simulink model "sim_3_twolink_task_control_ideal"  (R2021a)
settings: Solver=ode15s  StartTime=0.0  StopTime=20  RelTol=1e-5  EnableMultiTasking=on
values from neighbouring files (symbols this model uses):
  b1 = 0.01    [sim_params.m]    (also in sim_params_force.m)
  b2 = 0.01    [sim_params.m]    (also in sim_params_force.m)
  D = [zeros(n); eye(n)]    [control_comparison_script.m]    (also in gen_twolink_ss.m = reshape([0.0,0.0,0.0,0.0,0.0,0.0,0.0,0.0],[4,2]))
  D_T_Q = D'*Q    [control_comparison_script.m]
  epsilon = 0.1    [control_comparison_script.m]
  g = 9.80665    [sim_params.m]    (also in sim_params_force.m)
  Kpp = place(A,B,p)    [control_comparison_script.m]
  L1x = 0.3    [sim_params.m]    (also in sim_params_force.m)
  L1y = 0.050    (= 0.05)    [sim_params.m]    (also in sim_params_force.m)
  L1z = 0.05    [sim_params.m]    (also in sim_params_force.m)
  L2x = 0.15    [sim_params.m]    (also in sim_params_force.m = 0.3)
  L2y = 0.05    [sim_params.m]    (also in sim_params_force.m)
  L2z = 0.05    [sim_params.m]    (also in sim_params_force.m)
  m1 = m1*1.25    [control_comparison_script.m]    (also in sim_params.m = 2.775; sim_params_force.m = 2.775)
  m2 = m2*1.25    [control_comparison_script.m]    (also in sim_params.m = 1.3875; sim_params_force.m = 2.775)
  param_dev = 15    [control_comparison_script.m]
  rho = [1;1]    [control_comparison_script.m]
  theta1_0 = 0    [sim_params.m]    (also in sim_params_force.m = 1.57079632679)
  theta1_dot_0 = 0    [sim_params.m]    (also in sim_params_force.m)
  theta2_0 = 0    [sim_params.m]    (also in sim_params_force.m = -1.57079632679)
  theta2_dot_0 = 0    [sim_params.m]    (also in sim_params_force.m)
undefined symbols (not defined in the file or in its folder): Kd, Kd_grav, Kd_inv, Ki, Kp, Kp_grav, Kp_inv, N, sigbuilder_block, X, Y, Z
libraries: pid_lib x12, sm_lib x11, nesl_utility x10, spsFirstOrderFilterLib x4, dspmtrx3 x1, simulink x1
(part 1 of 3)
settings Model: Creator=bhorton  LastModifiedBy=Petronas-Tareq
settings SolverCC: ZeroCrossAlgorithm=Adaptive  AlgebraicLoopSolver=TrustRegion
settings DataIOCC: ReturnWorkspaceOutputs=off
settings OptimizationCC: LifeSpan=inf
settings DebuggingCC: SFUnexpectedBacktrackingDiag=warning  SFNoUnconditionalDefaultTransitionDiag=warning  SFExecutionAtInitializationDiag=none  SFMachineParentedDataDiag=warning  ArithmeticOperatorsInVariantConditions=warning
settings SFSimCC: SimUseLocalCustomCode=off  CustomCodeUndefinedFunction=UseInterfaceOnly
settings RTWCC: RTWUseLocalCustomCode=off
settings CodeAppCC: StateflowObjectComments=on
settings GRTTargetCC: TargetLangStandard=C89/C90 (ANSI)
settings ConfigComp: CovMetricSettings=dw  CovSaveCumulativeToWorkspaceVar=on  CovSaveSingleToWorkspaceVar=on  CovExternalEMLEnable=off
settings SimscapeCC: SimscapeNormalizeSystem=off  SimscapeLogType=all  SimscapeLogDataHistory=10000
settings ExplorerConfigSet: InternalSimMechanicsExplorerSettings="<ExplorerConfiguration><canonicalview>planar_xy</canonicalview><AnimationSetting><BasePlaybackSpeed>1.0</BasePlaybackSpeed><PlaybackSpeedFactor>4.0</PlaybackSpeedFactor></AnimationSetting><TilePanel><TileInfo><Tiles Columns=\"1\" Count=\"1\" Rows=\"1\"><Column Weight=\"1\"/><Row Weight=\"1\"/><Tile Height=\"1\" Width=\"1\" X=\"0\" Y=\"0\"/></Tiles></TileInfo><SceneInfo><SceneViewer><BGColor><R>0</R><G>0</G><B>0</B></BGColor><Camera><DoPerspective>off</DoPerspective><Position><X>0.0447898824465682299</X><Y>-0.016656403258507535</Y><Z>0.999999954328562035</Z></Position><Center><X>0.0447898824465682299</X><Y>-0.016656403258507535</Y><Z>-4.56714379648559543e-08</Z></Center><Up><X>0</X><Y>1</Y><Z>0</Z></Up><ViewLimDist>1</ViewLimDist><YLim>0.67213509984740738</YLim><XLim>1.22520332234454554</XLim></Camera></SceneViewer></SceneInfo></TilePanel><MechEditorPanel><Cameras/><GfxPanelCameraMap/><VideoCreator><PlaybackSpeedRatio>1</PlaybackSpeedRatio><FrameRate>30</FrameRate><VideoFormat>Motion JPEG AVI</VideoFormat><FrameSize>auto</FrameSize></VideoCreator></MechEditorPanel></ExplorerConfiguration>"

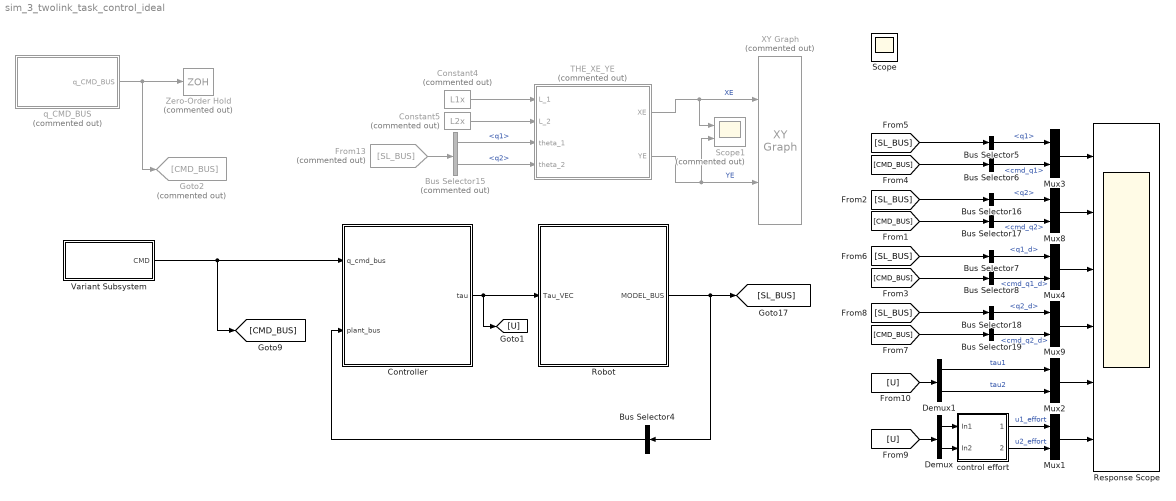
== system sim_3_twolink_task_control_ideal ==
  Bus Selector15 : BusSelector  Commented=on  OutputSignals=q1,q2
  Bus Selector16 : BusSelector  OutputSignals=q2
  Bus Selector17 : BusSelector  OutputSignals=cmd_q2
  Bus Selector18 : BusSelector  OutputSignals=q2_d
  Bus Selector19 : BusSelector  OutputSignals=cmd_q2_d
  Bus Selector4 : BusSelector  OutputSignals=q1_dd,q2_dd,q1_d,q2_d,q1,q2  OutputAsBus=on
  Bus Selector5 : BusSelector  OutputSignals=q1
  Bus Selector6 : BusSelector  OutputSignals=cmd_q1
  Bus Selector7 : BusSelector  OutputSignals=q1_d
  Bus Selector8 : BusSelector  OutputSignals=cmd_q1_d
  Constant4 : Constant  Commented=on  Value=L1x
  Constant5 : Constant  Commented=on  Value=L2x
  Controller : Subsystem  Variant=on  VariantControlMode=label  LabelModeActiveChoice=Inverse_dynamics_control  PropagateVariantConditions=on
  Demux : Demux  Outputs=2
  Demux1 : Demux  Outputs=2
  From13 : From  Commented=on  GotoTag=SL_BUS
  Goto2 : Goto  Commented=on  GotoTag=CMD_BUS
  Mux{1..4,8..9} (6 alike) : Mux  Inputs=2
  Response Scope : Scope  NumInputPorts=6
  Robot : Subsystem  Variant=on  VariantControlMode=label  LabelModeActiveChoice=Choice
  Scope1 : Scope  Commented=on  NumInputPorts=2
  THE_XE_YE : MATLAB Function  Commented=on  TreatAsAtomicUnit=on
  Variant Subsystem : Subsystem  Variant=on  VariantControlMode=label  LabelModeActiveChoice=Trapezoidal velocity
  XY Graph : simulink/Sinks/XY Graph  Commented=on  xmin=0  xmax=1.6  ymin=0  ymax=1.6  st=-1
  Zero-Order Hold : ZeroOrderHold  Commented=on  SampleTime=0.01
  control effort : Subsystem
  q_CMD_BUS : Subsystem  Commented=on
  Scope : Scope
  wires:
  [CMD_BUS] -> Bus Selector6/1
  [SL_BUS] -> Bus Selector5/1
  Mux3/1 -> Response Scope/1
  Bus Selector6/1 -> Mux3/2  "<cmd_q1>"
  Bus Selector5/1 -> Mux3/1  "<q1>"
  Bus Selector4/1 -> Controller/2(plant_bus)
  Mux4/1 -> Response Scope/3
  [SL_BUS] -> Bus Selector7/1
  [CMD_BUS] -> Bus Selector8/1
  Bus Selector8/1 -> Mux4/2  "<cmd_q1_d>"
  Bus Selector7/1 -> Mux4/1  "<q1_d>"
  Mux8/1 -> Response Scope/2
  [SL_BUS] -> Bus Selector16/1
  Bus Selector16/1 -> Mux8/1  "<q2>"
  [CMD_BUS] -> Bus Selector17/1
  Bus Selector17/1 -> Mux8/2  "<cmd_q2>"
  [CMD_BUS] -> Bus Selector19/1
  Mux9/1 -> Response Scope/4
  Bus Selector19/1 -> Mux9/2  "<cmd_q2_d>"
  Bus Selector18/1 -> Mux9/1  "<q2_d>"
  [SL_BUS] -> Bus Selector18/1
  Controller/1(tau) -> Robot/1(Tau_VEC), [U]
  [U] -> Demux/1
  Mux1/1 -> Response Scope/6
  Demux/1 -> control effort/1(In1)
  Demux/2 -> control effort/2(In2)
  control effort/1(u1_effort) -> Mux1/1  "u1_effort"
  control effort/2(u2_effort) -> Mux1/2  "u2_effort"
  [U] -> Demux1/1
  Mux2/1 -> Response Scope/5
  Demux1/1 -> Mux2/1  "tau1"
  Demux1/2 -> Mux2/2  "tau2"
  Variant Subsystem/1(CMD) -> [CMD_BUS], Controller/1(q_cmd_bus)
  Robot/1(MODEL_BUS) -> [SL_BUS], Bus Selector4/1
  From13/1 -> Bus Selector15/1
  Bus Selector15/2 -> THE_XE_YE/4(theta_2)  "<q2>"
  THE_XE_YE/2(YE) -> Scope1/2, XY Graph/2  "YE"
  Constant5/1 -> THE_XE_YE/2(L_2)
  Constant4/1 -> THE_XE_YE/1(L_1)
  THE_XE_YE/1(XE) -> Scope1/1, XY Graph/1  "XE"
  q_CMD_BUS/1(q_CMD_BUS) -> Goto2/1, Zero-Order Hold/1
  Bus Selector15/1 -> THE_XE_YE/3(theta_1)  "<q1>"

== system sim_3_twolink_task_control_ideal/Controller ==
  note: 1) Add Subsystem or Model blocks as valid variant choices.
      | 2) You cannot connect blocks at this level. At simulation, connectivity is automatically
      | determined, based on the active variant and port name matching.
  q_cmd_bus : Inport
  plant_bus : Inport  Port=2
  " Pole Placement Control" : Subsystem  VariantControl=PolePlacement_control
  "Inverse Dynamics control " : Subsystem  VariantControl=Inverse_dynamics_control
  PD Control : Subsystem  VariantControl=PD_control
  PD-feedforward-gravity Control : Subsystem  VariantControl=PD_feedforward_gravity
  "PD-gravity Control " : Subsystem  VariantControl=PD_plus_gravity
  PID Control : Subsystem  VariantControl=PID_control
  Pole Placement+D Control : Subsystem  VariantControl=PolePlacement_D_control
  "Robust control " : Subsystem  VariantControl=robust_control
  tau : Outport

== system sim_3_twolink_task_control_ideal/Robot ==
  note: 1) Add Subsystem or Model blocks as valid variant choices.
      | 2) You cannot connect blocks at this level. At simulation, connectivity is automatically
      | determined, based on the active variant and port name matching.
  Tau_VEC : Inport
  SIMSCAPE_MODEL : Subsystem  VariantControl=Choice_1
  SIMULINK_MODEL : Subsystem  VariantControl=Choice
  MODEL_BUS : Outport

== system sim_3_twolink_task_control_ideal/Variant Subsystem ==
  note: 1) Add Subsystem or Model blocks as valid variant choices.
      | 2) You cannot connect blocks at this level. At simulation, connectivity is automatically
      | determined, based on the active variant and port name matching.
  Sinewave command : Subsystem  VariantControl=sinwave
  Step command : Subsystem  VariantControl=step
  Trapezoidal velocity : Subsystem  VariantControl=Trapezoidal velocity
  CMD : Outport

== system sim_3_twolink_task_control_ideal/control effort ==
  In1 : Inport
  In2 : Inport  Port=2
  Integrator : Integrator
  Integrator1 : Integrator
  Square : Math  Operator=square  SaturateOnIntegerOverflow=on
  Square1 : Math  Operator=square  SaturateOnIntegerOverflow=on
  u1_effort : Outport
  u2_effort : Outport  Port=2
  wires:
  Square/1 -> Integrator/1
  Integrator1/1 -> u2_effort/1  "u2_effort"
  Integrator/1 -> u1_effort/1  "u1_effort"
  Square1/1 -> Integrator1/1
  In2/1 -> Square1/1
  In1/1 -> Square/1

== system sim_3_twolink_task_control_ideal/q_CMD_BUS ==
  Bus Creator : BusCreator  Inputs=4
  Bus Selector : BusSelector  OutputSignals=cmd_q1_d,cmd_q2_d,cmd_q1,cmd_q2
  From Spreadsheet : FromSpreadsheet  FileName=bh_2dof_q1_q2_for_hello.xlsx  SheetName=Q_for_hello  SampleTime=-1  ExtrapolationBeforeFirstDataPoint=Hold first value  ExtrapolationAfterLastDataPoint=Hold last value
  Scope : Scope  NumInputPorts=4
  q_CMD_BUS : Outport
  wires:
  From Spreadsheet/2 -> Bus Creator/2  "cmd_q2_d"
  From Spreadsheet/3 -> Bus Creator/3  "cmd_q1"
  From Spreadsheet/1 -> Bus Creator/1  "cmd_q1_d"
  From Spreadsheet/4 -> Bus Creator/4  "cmd_q2"
  Bus Creator/1 -> Bus Selector/1, q_CMD_BUS/1
  Bus Selector/1 -> Scope/1  "<cmd_q1_d>"
  Bus Selector/2 -> Scope/2  "<cmd_q2_d>"
  Bus Selector/3 -> Scope/3  "<cmd_q1>"
  Bus Selector/4 -> Scope/4  "<cmd_q2>"

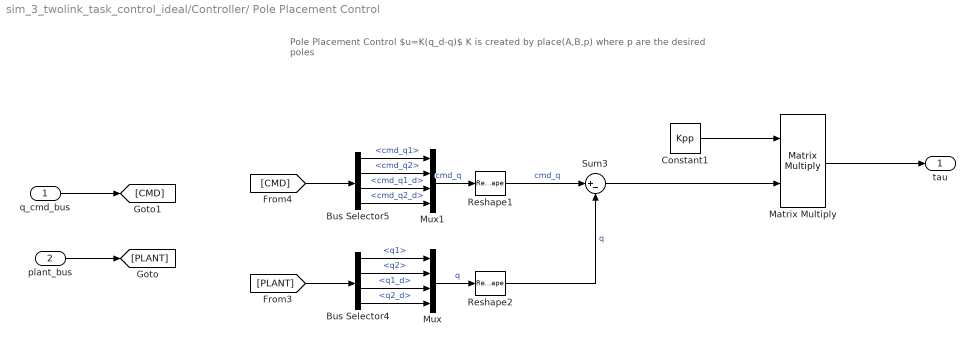
== system sim_3_twolink_task_control_ideal/Controller/ Pole Placement Control ==
  note: Pole Placement Control
      | $u=K(q_d-q)$
      | K is created by place(A,B,p) where p are the desired poles
  q_cmd_bus : Inport
  plant_bus : Inport  Port=2
  Bus Selector4 : BusSelector  OutputSignals=q1,q2,q1_d,q2_d
  Bus Selector5 : BusSelector  OutputSignals=cmd_q1,cmd_q2,cmd_q1_d,cmd_q2_d
  Constant1 : Constant  Value=Kpp  VectorParams1D=off
  Matrix Multiply : Product  Multiplication=Matrix(*)
  Mux : Mux
  Mux1 : Mux
  Reshape1 : Reshape  OutputDimensionality=Column vector (2-D)
  Reshape2 : Reshape  OutputDimensionality=Column vector (2-D)
  Sum3 : Sum  Inputs=|+-
  tau : Outport
  wires:
  plant_bus/1 -> [PLANT]
  q_cmd_bus/1 -> [CMD]
  [PLANT] -> Bus Selector4/1
  Bus Selector4/3 -> Mux/3  "<q1_d>"
  Bus Selector4/4 -> Mux/4  "<q2_d>"
  Mux/1 -> Reshape2/1  "q"
  Mux1/1 -> Reshape1/1  "cmd_q"
  [CMD] -> Bus Selector5/1
  Bus Selector5/3 -> Mux1/3  "<cmd_q1_d>"
  Bus Selector5/4 -> Mux1/4  "<cmd_q2_d>"
  Bus Selector5/2 -> Mux1/2  "<cmd_q2>"
  Bus Selector5/1 -> Mux1/1  "<cmd_q1>"
  Sum3/1 -> Matrix Multiply/2
  Reshape2/1 -> Sum3/2  "q"
  Reshape1/1 -> Sum3/1  "cmd_q"
  Constant1/1 -> Matrix Multiply/1
  Bus Selector4/1 -> Mux/1  "<q1>"
  Bus Selector4/2 -> Mux/2  "<q2>"
  Matrix Multiply/1 -> tau/1

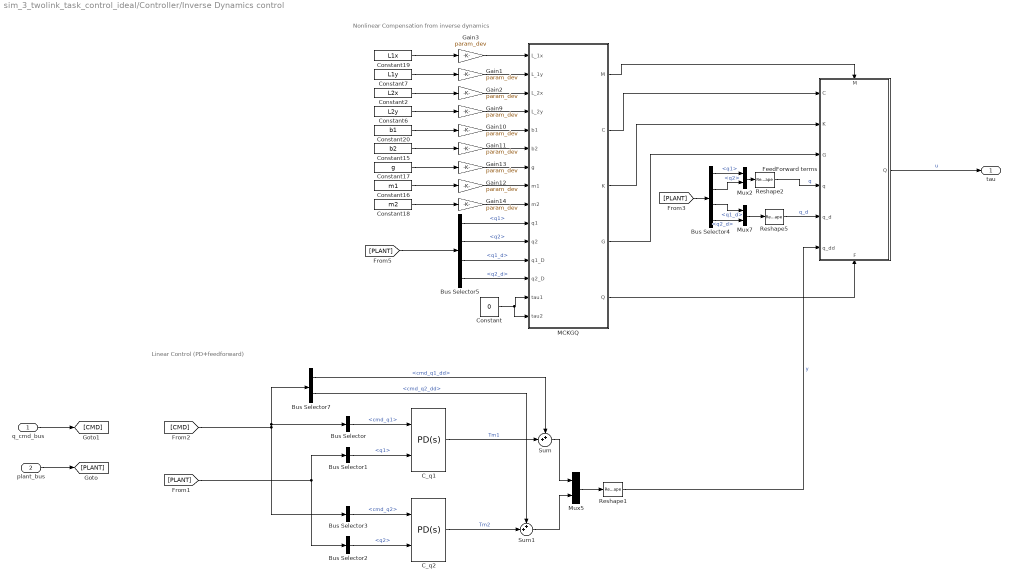
== system sim_3_twolink_task_control_ideal/Controller/Inverse Dynamics control  ==
  note: Nonlinear Compensation from inverse dynamics
  note: Linear Control (PD+feedforward)
  q_cmd_bus : Inport
  plant_bus : Inport  Port=2
  Bus Selector : BusSelector  OutputSignals=cmd_q1
  Bus Selector1 : BusSelector  OutputSignals=q1
  Bus Selector2 : BusSelector  OutputSignals=q2
  Bus Selector3 : BusSelector  OutputSignals=cmd_q2
  Bus Selector4 : BusSelector  OutputSignals=q1,q2,q1_d,q2_d
  Bus Selector5 : BusSelector  OutputSignals=q1,q2,q1_d,q2_d
  Bus Selector7 : BusSelector  OutputSignals=cmd_q1_dd,cmd_q2_dd
  C_q1 : pid_lib/PID Controller (2DOF)  Controller=PD  Form=Parallel  TimeDomain=Continuous-time  UseExternalTs=off  SampleTime=-1  IntegratorMethod=Forward Euler  FilterMethod=Forward Euler  ControllerParametersSource=internal  P=Kp_inv  I=20  D=Kd_inv  UseFilter=on  N=N  b=1  c=1  TunerSelectOption=Transfer Function Based (PID Tuner App)  InitialConditionSource=internal  InitialConditionForIntegrator=0  InitialConditionForFilter=0  DifferentiatorICPrevScaledInput=0  ExternalReset=none  TrackingMode=off  Kt=1  LimitOutput=off  SatLimitsSource=internal  UpperSaturationLimit=inf  LowerSaturationLimit=-inf  LinearizeAsGain=on  AntiWindupMode=none  Kb=1  POutMin=[]  POutMax=[]  IOutMin=[]  IOutMax=[]  DOutMin=[]  DOutMax=[]  NOutMin=[]  NOutMax=[]  bOutMin=[]  bOutMax=[]  cOutMin=[]  cOutMax=[]  SumOutMin=[]  SumOutMax=[]  SaturationOutMin=[]  SaturationOutMax=[]  PParamMin=[]  PParamMax=[]  IParamMin=[]  IParamMax=[]  DParamMin=[]  DParamMax=[]  NParamMin=[]  NParamMax=[]  bParamMin=[]  bParamMax=[]  cParamMin=[]  cParamMax=[]  KbParamMin=[]  KbParamMax=[]  KtParamMin=[]  KtParamMax=[]  KbOutMin=[]  KbOutMax=[]  KtOutMin=[]  KtOutMax=[]  IntegratorOutMin=[]  IntegratorOutMax=[]  FilterOutMin=[]  FilterOutMax=[]  SumI1OutMin=[]  SumI1OutMax=[]  SumI2OutMin=[]  SumI2OutMax=[]  SumI3OutMin=[]  SumI3OutMax=[]  SumI4OutMin=[]  SumI4OutMax=[]  SumDOutMin=[]  SumDOutMax=[]  Sum1OutMin=[]  Sum1OutMax=[]  Sum2OutMin=[]  Sum2OutMax=[]  Sum3OutMin=[]  Sum3OutMax=[]  DifferentiatorOutMin=[]  DifferentiatorOutMax=[]  FilterDiffOutCoefMin=[]  FilterDiffOutCoefMax=[]  ReciprocalOutMin=[]  ReciprocalOutMax=[]  SumDenOutMin=[]  SumDenOutMax=[]  SumNumOutMin=[]  SumNumOutMax=[]  DivideOutMin=[]  DivideOutMax=[]  UdiffTsProdOutMin=[]  UdiffTsProdOutMax=[]  NTsProdOutMin=[]  NTsProdOutMax=[]  UintegralTsProdOutMin=[]  UintegralTsProdOutMax=[]  UngainTsProdOutMin=[]  UngainTsProdOutMax=[]  IntegratorContinuousStateAttributes=''  IntegratorStateMustResolveToSignalObject=off  IntegratorRTWStateStorageClass=Auto  FilterContinuousStateAttributes=''  FilterStateMustResolveToSignalObject=off  FilterRTWStateStorageClass=Auto  ParallelPVariant=InternalParameters  IdealPVariant=Disabled  IVariant=Disabled  DVariant=InternalParameters  bVariant=InternalParameters  cVariant=InternalParameters  IntegratorVariant=Disabled  SatVariant=Disabled  AWVariant=Disabled  PCopyVariant=Disabled  TRVariant=Disabled  FdbkBlocksVariant=Forward  IdealPFdbkVariant=Disabled  SatFdbkVariant=Disabled  DerivativeFilterVariant=ContFilter  NVariant=InternalParameters  NCopyVariant=Disabled  FilterICVariant=InternalICsFilter  IntegratorICVariant=Disabled  ExternalResetVariant=Disabled  TRSumVariant=Passthrough  SumFdbkVariant=Disabled  SumVariant=Sum_PD  TsampFilterVariant=InternalTs  TsampNgainVariant=Passthrough  TsampIntegralVariant=Disabled_SignalSpec  ExternalSaturationOutDataTypeStr=Inherit: Same as second input
      settings: SourceProductBaseCode=SL
  C_q2 : pid_lib/PID Controller (2DOF)  Controller=PD  Form=Parallel  TimeDomain=Continuous-time  UseExternalTs=off  SampleTime=-1  IntegratorMethod=Forward Euler  FilterMethod=Forward Euler  ControllerParametersSource=internal  P=Kp_inv  I=20  D=Kd_inv  UseFilter=on  N=N  b=1  c=1  TunerSelectOption=Transfer Function Based (PID Tuner App)  InitialConditionSource=internal  InitialConditionForIntegrator=0  InitialConditionForFilter=0  DifferentiatorICPrevScaledInput=0  ExternalReset=none  TrackingMode=off  Kt=1  LimitOutput=off  SatLimitsSource=internal  UpperSaturationLimit=inf  LowerSaturationLimit=-inf  LinearizeAsGain=on  AntiWindupMode=none  Kb=1  POutMin=[]  POutMax=[]  IOutMin=[]  IOutMax=[]  DOutMin=[]  DOutMax=[]  NOutMin=[]  NOutMax=[]  bOutMin=[]  bOutMax=[]  cOutMin=[]  cOutMax=[]  SumOutMin=[]  SumOutMax=[]  SaturationOutMin=[]  SaturationOutMax=[]  PParamMin=[]  PParamMax=[]  IParamMin=[]  IParamMax=[]  DParamMin=[]  DParamMax=[]  NParamMin=[]  NParamMax=[]  bParamMin=[]  bParamMax=[]  cParamMin=[]  cParamMax=[]  KbParamMin=[]  KbParamMax=[]  KtParamMin=[]  KtParamMax=[]  KbOutMin=[]  KbOutMax=[]  KtOutMin=[]  KtOutMax=[]  IntegratorOutMin=[]  IntegratorOutMax=[]  FilterOutMin=[]  FilterOutMax=[]  SumI1OutMin=[]  SumI1OutMax=[]  SumI2OutMin=[]  SumI2OutMax=[]  SumI3OutMin=[]  SumI3OutMax=[]  SumI4OutMin=[]  SumI4OutMax=[]  SumDOutMin=[]  SumDOutMax=[]  Sum1OutMin=[]  Sum1OutMax=[]  Sum2OutMin=[]  Sum2OutMax=[]  Sum3OutMin=[]  Sum3OutMax=[]  DifferentiatorOutMin=[]  DifferentiatorOutMax=[]  FilterDiffOutCoefMin=[]  FilterDiffOutCoefMax=[]  ReciprocalOutMin=[]  ReciprocalOutMax=[]  SumDenOutMin=[]  SumDenOutMax=[]  SumNumOutMin=[]  SumNumOutMax=[]  DivideOutMin=[]  DivideOutMax=[]  UdiffTsProdOutMin=[]  UdiffTsProdOutMax=[]  NTsProdOutMin=[]  NTsProdOutMax=[]  UintegralTsProdOutMin=[]  UintegralTsProdOutMax=[]  UngainTsProdOutMin=[]  UngainTsProdOutMax=[]  IntegratorContinuousStateAttributes=''  IntegratorStateMustResolveToSignalObject=off  IntegratorRTWStateStorageClass=Auto  FilterContinuousStateAttributes=''  FilterStateMustResolveToSignalObject=off  FilterRTWStateStorageClass=Auto  ParallelPVariant=InternalParameters  IdealPVariant=Disabled  IVariant=Disabled  DVariant=InternalParameters  bVariant=InternalParameters  cVariant=InternalParameters  IntegratorVariant=Disabled  SatVariant=Disabled  AWVariant=Disabled  PCopyVariant=Disabled  TRVariant=Disabled  FdbkBlocksVariant=Forward  IdealPFdbkVariant=Disabled  SatFdbkVariant=Disabled  DerivativeFilterVariant=ContFilter  NVariant=InternalParameters  NCopyVariant=Disabled  FilterICVariant=InternalICsFilter  IntegratorICVariant=Disabled  ExternalResetVariant=Disabled  TRSumVariant=Passthrough  SumFdbkVariant=Disabled  SumVariant=Sum_PD  TsampFilterVariant=InternalTs  TsampNgainVariant=Passthrough  TsampIntegralVariant=Disabled_SignalSpec  ExternalSaturationOutDataTypeStr=Inherit: Same as second input
      settings: SourceProductBaseCode=SL
  Constant : Constant  Value=0
  Constant15 : Constant  Value=b2
  Constant16 : Constant  Value=m1
  Constant17 : Constant  Value=g
  Constant18 : Constant  Value=m2
  Constant19 : Constant  Value=L1x
  Constant2 : Constant  Value=L2x
  Constant20 : Constant  Value=b1
  Constant6 : Constant  Value=L2y
  Constant7 : Constant  Value=L1y
  FeedForward terms : Subsystem
      settings: PortSchema="{\"entries\":[{\"content\":{\"sides\":[{\"content\":{\"connectorIds\":[\"In1\",\"In2\",\"In3\",\"In4\",\"In5\",\"In6\"]},\"type\":\"ConnectorPlacement.EquallySpacedRectSide\",\"uuid\":\"236e7a2f-027c-4887-b3e9-bc0e11a59ec6\"},{\"content\":{\"connectorIds\":[\"Out1\"],\"side\":\"RIGHT\"},\"type\":\"ConnectorPlacement.EquallySpacedRectSide\",\"uuid\":\"0b727d96-7650-4ea0-95ac-5fb1bad7af10\"},{\"content\":{\"connectorIds\":[\"In7\"],\"side\":\"TOP\"},\"type\":\"ConnectorPlacement.EquallySpacedRectSide\",\"uuid\":\"19d9c8c6-ae7e-49b4-b718-472bd3040569\"},{\"content\":{\"connectorIds\":[\"In8\"],\"side\":\"BOTTOM\"},\"type\":\"ConnectorPlacement.EquallySpacedRectSide\",\"uuid\":\"734f5953-872d-4718-8798-69ea98da43e1\"}]},\"type\":\"ConnectorPlacement.EquallySpacedConnector\",\"uuid\":\"f4b93fea-e2dd-47f1-bf2a-cf2dec03adb9\"}],\"packageUris\":[\"http://schema.mathworks.com/mf0/Connector/R2020b\"],\"version\":\"1.0\"}"
  Gain{1..3,9..14} (9 alike) : Gain  Gain=param_dev
  MCKGQ : MATLAB Function  TreatAsAtomicUnit=on
  Mux2 : Mux  Inputs=2
  Mux5 : Mux  Inputs=2
  Mux7 : Mux  Inputs=2
  Reshape1 : Reshape  OutputDimensionality=Column vector (2-D)
  Reshape2 : Reshape  OutputDimensionality=Column vector (2-D)
  Reshape5 : Reshape  OutputDimensionality=Column vector (2-D)
  Sum : Sum  Inputs=++|
  Sum1 : Sum  Inputs=++|
  tau : Outport
  wires:
  C_q1/1 -> Sum/2  "Tm1"
  q_cmd_bus/1 -> [CMD]
  plant_bus/1 -> [PLANT]
  Bus Selector2/1 -> C_q2/2  "<q2>"
  Bus Selector3/1 -> C_q2/1  "<cmd_q2>"
  Bus Selector1/1 -> C_q1/2  "<q1>"
  Bus Selector/1 -> C_q1/1  "<cmd_q1>"
  [PLANT] -> Bus Selector1/1, Bus Selector2/1
  Constant17/1 -> Gain13/1
  Bus Selector5/4 -> MCKGQ/13(q2_D)  "<q2_d>"
  Constant16/1 -> Gain12/1
  Constant20/1 -> Gain10/1
  Constant2/1 -> Gain2/1
  Bus Selector5/3 -> MCKGQ/12(q1_D)  "<q1_d>"
  Bus Selector5/1 -> MCKGQ/10(q1)  "<q1>"
  Constant19/1 -> Gain3/1
  Constant15/1 -> Gain11/1
  Constant6/1 -> Gain9/1
  Constant7/1 -> Gain1/1
  Constant18/1 -> Gain14/1
  [PLANT] -> Bus Selector5/1
  Bus Selector5/2 -> MCKGQ/11(q2)  "<q2>"
  Mux5/1 -> Reshape1/1
  FeedForward terms/1(Q) -> tau/1  "u"
  [CMD] -> Bus Selector7/1, Bus Selector/1, Bus Selector3/1
  Bus Selector7/2 -> Sum1/1  "<cmd_q2_dd>"
  Sum/1 -> Mux5/1
  C_q2/1 -> Sum1/2  "Tm2"
  Sum1/1 -> Mux5/2
  [PLANT] -> Bus Selector4/1
  Bus Selector4/3 -> Mux7/1  "<q1_d>"
  Bus Selector4/4 -> Mux7/2  "<q2_d>"
  Mux7/1 -> Reshape5/1
  Reshape5/1 -> FeedForward terms/5(q_d)  "q_d"
  Reshape1/1 -> FeedForward terms/6(q_dd)  "y"
  MCKGQ/2(C) -> FeedForward terms/1(C)
  MCKGQ/3(K) -> FeedForward terms/2(K)
  MCKGQ/4(G) -> FeedForward terms/3(G)
  Bus Selector4/1 -> Mux2/1  "<q1>"
  Bus Selector4/2 -> Mux2/2  "<q2>"
  Mux2/1 -> Reshape2/1
  Reshape2/1 -> FeedForward terms/4(q)  "q"
  Bus Selector7/1 -> Sum/1  "<cmd_q1_dd>"
  MCKGQ/5(Q) -> FeedForward terms/8(F)
  Constant/1 -> MCKGQ/14(tau1), MCKGQ/15(tau2)
  MCKGQ/1(M) -> FeedForward terms/7(M)
  Gain1/1 -> MCKGQ/2(L_1y)
  Gain2/1 -> MCKGQ/3(L_2x)
  Gain9/1 -> MCKGQ/4(L_2y)
  Gain10/1 -> MCKGQ/5(b1)
  Gain11/1 -> MCKGQ/6(b2)
  Gain13/1 -> MCKGQ/7(g)
  Gain12/1 -> MCKGQ/8(m1)
  Gain14/1 -> MCKGQ/9(m2)
  Gain3/1 -> MCKGQ/1(L_1x)

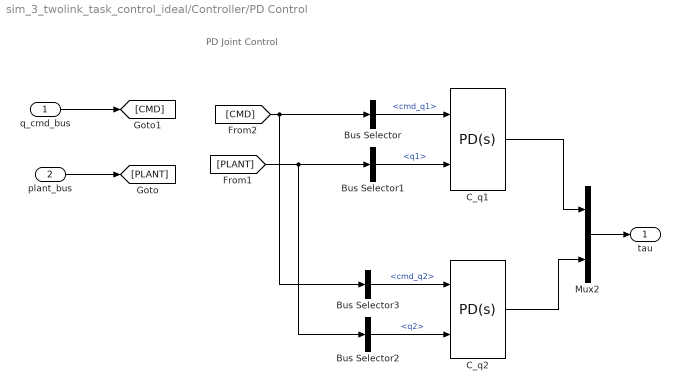
== system sim_3_twolink_task_control_ideal/Controller/PD Control ==
  note: PD Joint Control
  q_cmd_bus : Inport
  plant_bus : Inport  Port=2
  Bus Selector : BusSelector  OutputSignals=cmd_q1
  Bus Selector1 : BusSelector  OutputSignals=q1
  Bus Selector2 : BusSelector  OutputSignals=q2
  Bus Selector3 : BusSelector  OutputSignals=cmd_q2
  C_q1 : pid_lib/PID Controller (2DOF)  Controller=PD  Form=Parallel  TimeDomain=Continuous-time  UseExternalTs=off  SampleTime=-1  IntegratorMethod=Forward Euler  FilterMethod=Forward Euler  ControllerParametersSource=internal  P=Kp  I=20  D=Kd  UseFilter=on  N=N  b=1  c=1  TunerSelectOption=Transfer Function Based (PID Tuner App)  InitialConditionSource=internal  InitialConditionForIntegrator=0  InitialConditionForFilter=0  DifferentiatorICPrevScaledInput=0  ExternalReset=none  TrackingMode=off  Kt=1  LimitOutput=off  SatLimitsSource=internal  UpperSaturationLimit=inf  LowerSaturationLimit=-inf  LinearizeAsGain=on  AntiWindupMode=none  Kb=1  POutMin=[]  POutMax=[]  IOutMin=[]  IOutMax=[]  DOutMin=[]  DOutMax=[]  NOutMin=[]  NOutMax=[]  bOutMin=[]  bOutMax=[]  cOutMin=[]  cOutMax=[]  SumOutMin=[]  SumOutMax=[]  SaturationOutMin=[]  SaturationOutMax=[]  PParamMin=[]  PParamMax=[]  IParamMin=[]  IParamMax=[]  DParamMin=[]  DParamMax=[]  NParamMin=[]  NParamMax=[]  bParamMin=[]  bParamMax=[]  cParamMin=[]  cParamMax=[]  KbParamMin=[]  KbParamMax=[]  KtParamMin=[]  KtParamMax=[]  KbOutMin=[]  KbOutMax=[]  KtOutMin=[]  KtOutMax=[]  IntegratorOutMin=[]  IntegratorOutMax=[]  FilterOutMin=[]  FilterOutMax=[]  SumI1OutMin=[]  SumI1OutMax=[]  SumI2OutMin=[]  SumI2OutMax=[]  SumI3OutMin=[]  SumI3OutMax=[]  SumI4OutMin=[]  SumI4OutMax=[]  SumDOutMin=[]  SumDOutMax=[]  Sum1OutMin=[]  Sum1OutMax=[]  Sum2OutMin=[]  Sum2OutMax=[]  Sum3OutMin=[]  Sum3OutMax=[]  DifferentiatorOutMin=[]  DifferentiatorOutMax=[]  FilterDiffOutCoefMin=[]  FilterDiffOutCoefMax=[]  ReciprocalOutMin=[]  ReciprocalOutMax=[]  SumDenOutMin=[]  SumDenOutMax=[]  SumNumOutMin=[]  SumNumOutMax=[]  DivideOutMin=[]  DivideOutMax=[]  UdiffTsProdOutMin=[]  UdiffTsProdOutMax=[]  NTsProdOutMin=[]  NTsProdOutMax=[]  UintegralTsProdOutMin=[]  UintegralTsProdOutMax=[]  UngainTsProdOutMin=[]  UngainTsProdOutMax=[]  IntegratorContinuousStateAttributes=''  IntegratorStateMustResolveToSignalObject=off  IntegratorRTWStateStorageClass=Auto  FilterContinuousStateAttributes=''  FilterStateMustResolveToSignalObject=off  FilterRTWStateStorageClass=Auto  ParallelPVariant=InternalParameters  IdealPVariant=Disabled  IVariant=Disabled  DVariant=InternalParameters  bVariant=InternalParameters  cVariant=InternalParameters  IntegratorVariant=Disabled  SatVariant=Disabled  AWVariant=Disabled  PCopyVariant=Disabled  TRVariant=Disabled  FdbkBlocksVariant=Forward  IdealPFdbkVariant=Disabled  SatFdbkVariant=Disabled  DerivativeFilterVariant=ContFilter  NVariant=InternalParameters  NCopyVariant=Disabled  FilterICVariant=InternalICsFilter  IntegratorICVariant=Disabled  ExternalResetVariant=Disabled  TRSumVariant=Passthrough  SumFdbkVariant=Disabled  SumVariant=Sum_PD  TsampFilterVariant=InternalTs  TsampNgainVariant=Passthrough  TsampIntegralVariant=Disabled_SignalSpec  ExternalSaturationOutDataTypeStr=Inherit: Same as second input
      settings: SourceProductBaseCode=SL
  C_q2 : pid_lib/PID Controller (2DOF)  Controller=PD  Form=Parallel  TimeDomain=Continuous-time  UseExternalTs=off  SampleTime=-1  IntegratorMethod=Forward Euler  FilterMethod=Forward Euler  ControllerParametersSource=internal  P=Kp  I=307.702571204868  D=Kd  UseFilter=on  N=N  b=1  c=1  TunerSelectOption=Transfer Function Based (PID Tuner App)  InitialConditionSource=internal  InitialConditionForIntegrator=0  InitialConditionForFilter=0  DifferentiatorICPrevScaledInput=0  ExternalReset=none  TrackingMode=off  Kt=1  LimitOutput=off  SatLimitsSource=internal  UpperSaturationLimit=inf  LowerSaturationLimit=-inf  LinearizeAsGain=on  AntiWindupMode=none  Kb=1  POutMin=[]  POutMax=[]  IOutMin=[]  IOutMax=[]  DOutMin=[]  DOutMax=[]  NOutMin=[]  NOutMax=[]  bOutMin=[]  bOutMax=[]  cOutMin=[]  cOutMax=[]  SumOutMin=[]  SumOutMax=[]  SaturationOutMin=[]  SaturationOutMax=[]  PParamMin=[]  PParamMax=[]  IParamMin=[]  IParamMax=[]  DParamMin=[]  DParamMax=[]  NParamMin=[]  NParamMax=[]  bParamMin=[]  bParamMax=[]  cParamMin=[]  cParamMax=[]  KbParamMin=[]  KbParamMax=[]  KtParamMin=[]  KtParamMax=[]  KbOutMin=[]  KbOutMax=[]  KtOutMin=[]  KtOutMax=[]  IntegratorOutMin=[]  IntegratorOutMax=[]  FilterOutMin=[]  FilterOutMax=[]  SumI1OutMin=[]  SumI1OutMax=[]  SumI2OutMin=[]  SumI2OutMax=[]  SumI3OutMin=[]  SumI3OutMax=[]  SumI4OutMin=[]  SumI4OutMax=[]  SumDOutMin=[]  SumDOutMax=[]  Sum1OutMin=[]  Sum1OutMax=[]  Sum2OutMin=[]  Sum2OutMax=[]  Sum3OutMin=[]  Sum3OutMax=[]  DifferentiatorOutMin=[]  DifferentiatorOutMax=[]  FilterDiffOutCoefMin=[]  FilterDiffOutCoefMax=[]  ReciprocalOutMin=[]  ReciprocalOutMax=[]  SumDenOutMin=[]  SumDenOutMax=[]  SumNumOutMin=[]  SumNumOutMax=[]  DivideOutMin=[]  DivideOutMax=[]  UdiffTsProdOutMin=[]  UdiffTsProdOutMax=[]  NTsProdOutMin=[]  NTsProdOutMax=[]  UintegralTsProdOutMin=[]  UintegralTsProdOutMax=[]  UngainTsProdOutMin=[]  UngainTsProdOutMax=[]  IntegratorContinuousStateAttributes=''  IntegratorStateMustResolveToSignalObject=off  IntegratorRTWStateStorageClass=Auto  FilterContinuousStateAttributes=''  FilterStateMustResolveToSignalObject=off  FilterRTWStateStorageClass=Auto  ParallelPVariant=InternalParameters  IdealPVariant=Disabled  IVariant=Disabled  DVariant=InternalParameters  bVariant=InternalParameters  cVariant=InternalParameters  IntegratorVariant=Disabled  SatVariant=Disabled  AWVariant=Disabled  PCopyVariant=Disabled  TRVariant=Disabled  FdbkBlocksVariant=Forward  IdealPFdbkVariant=Disabled  SatFdbkVariant=Disabled  DerivativeFilterVariant=ContFilter  NVariant=InternalParameters  NCopyVariant=Disabled  FilterICVariant=InternalICsFilter  IntegratorICVariant=Disabled  ExternalResetVariant=Disabled  TRSumVariant=Passthrough  SumFdbkVariant=Disabled  SumVariant=Sum_PD  TsampFilterVariant=InternalTs  TsampNgainVariant=Passthrough  TsampIntegralVariant=Disabled_SignalSpec  ExternalSaturationOutDataTypeStr=Inherit: Same as second input
      settings: SourceProductBaseCode=SL
  Mux2 : Mux  Inputs=2
  tau : Outport
  wires:
  [CMD] -> Bus Selector3/1, Bus Selector/1
  [PLANT] -> Bus Selector2/1, Bus Selector1/1
  Bus Selector/1 -> C_q1/1  "<cmd_q1>"
  Bus Selector1/1 -> C_q1/2  "<q1>"
  Bus Selector3/1 -> C_q2/1  "<cmd_q2>"
  Bus Selector2/1 -> C_q2/2  "<q2>"
  plant_bus/1 -> [PLANT]
  q_cmd_bus/1 -> [CMD]
  C_q2/1 -> Mux2/2
  C_q1/1 -> Mux2/1
  Mux2/1 -> tau/1

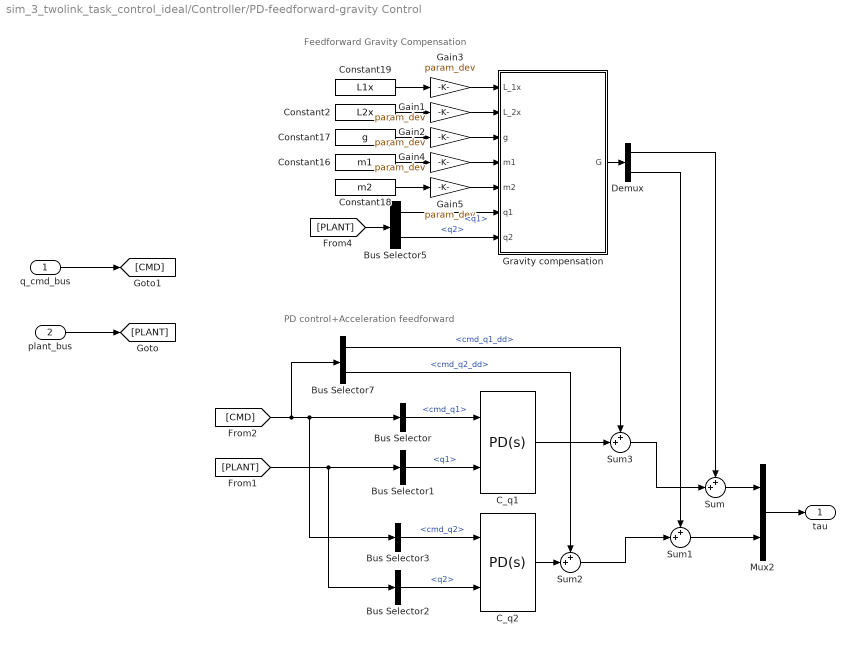
== system sim_3_twolink_task_control_ideal/Controller/PD-feedforward-gravity Control ==
  note: PD control+Acceleration feedforward
  note: Feedforward Gravity Compensation
  q_cmd_bus : Inport
  plant_bus : Inport  Port=2
  Bus Selector : BusSelector  OutputSignals=cmd_q1
  Bus Selector1 : BusSelector  OutputSignals=q1
  Bus Selector2 : BusSelector  OutputSignals=q2
  Bus Selector3 : BusSelector  OutputSignals=cmd_q2
  Bus Selector5 : BusSelector  OutputSignals=q1,q2
  Bus Selector7 : BusSelector  OutputSignals=cmd_q1_dd,cmd_q2_dd
  C_q1 : pid_lib/PID Controller (2DOF)  Controller=PD  Form=Parallel  TimeDomain=Continuous-time  UseExternalTs=off  SampleTime=-1  IntegratorMethod=Forward Euler  FilterMethod=Forward Euler  ControllerParametersSource=internal  P=Kp_grav  I=20  D=Kd_grav  UseFilter=on  N=N  b=1  c=1  TunerSelectOption=Transfer Function Based (PID Tuner App)  InitialConditionSource=internal  InitialConditionForIntegrator=0  InitialConditionForFilter=0  DifferentiatorICPrevScaledInput=0  ExternalReset=none  TrackingMode=off  Kt=1  LimitOutput=off  SatLimitsSource=internal  UpperSaturationLimit=inf  LowerSaturationLimit=-inf  LinearizeAsGain=on  AntiWindupMode=none  Kb=1  POutMin=[]  POutMax=[]  IOutMin=[]  IOutMax=[]  DOutMin=[]  DOutMax=[]  NOutMin=[]  NOutMax=[]  bOutMin=[]  bOutMax=[]  cOutMin=[]  cOutMax=[]  SumOutMin=[]  SumOutMax=[]  SaturationOutMin=[]  SaturationOutMax=[]  PParamMin=[]  PParamMax=[]  IParamMin=[]  IParamMax=[]  DParamMin=[]  DParamMax=[]  NParamMin=[]  NParamMax=[]  bParamMin=[]  bParamMax=[]  cParamMin=[]  cParamMax=[]  KbParamMin=[]  KbParamMax=[]  KtParamMin=[]  KtParamMax=[]  KbOutMin=[]  KbOutMax=[]  KtOutMin=[]  KtOutMax=[]  IntegratorOutMin=[]  IntegratorOutMax=[]  FilterOutMin=[]  FilterOutMax=[]  SumI1OutMin=[]  SumI1OutMax=[]  SumI2OutMin=[]  SumI2OutMax=[]  SumI3OutMin=[]  SumI3OutMax=[]  SumI4OutMin=[]  SumI4OutMax=[]  SumDOutMin=[]  SumDOutMax=[]  Sum1OutMin=[]  Sum1OutMax=[]  Sum2OutMin=[]  Sum2OutMax=[]  Sum3OutMin=[]  Sum3OutMax=[]  DifferentiatorOutMin=[]  DifferentiatorOutMax=[]  FilterDiffOutCoefMin=[]  FilterDiffOutCoefMax=[]  ReciprocalOutMin=[]  ReciprocalOutMax=[]  SumDenOutMin=[]  SumDenOutMax=[]  SumNumOutMin=[]  SumNumOutMax=[]  DivideOutMin=[]  DivideOutMax=[]  UdiffTsProdOutMin=[]  UdiffTsProdOutMax=[]  NTsProdOutMin=[]  NTsProdOutMax=[]  UintegralTsProdOutMin=[]  UintegralTsProdOutMax=[]  UngainTsProdOutMin=[]  UngainTsProdOutMax=[]  IntegratorContinuousStateAttributes=''  IntegratorStateMustResolveToSignalObject=off  IntegratorRTWStateStorageClass=Auto  FilterContinuousStateAttributes=''  FilterStateMustResolveToSignalObject=off  FilterRTWStateStorageClass=Auto  ParallelPVariant=InternalParameters  IdealPVariant=Disabled  IVariant=Disabled  DVariant=InternalParameters  bVariant=InternalParameters  cVariant=InternalParameters  IntegratorVariant=Disabled  SatVariant=Disabled  AWVariant=Disabled  PCopyVariant=Disabled  TRVariant=Disabled  FdbkBlocksVariant=Forward  IdealPFdbkVariant=Disabled  SatFdbkVariant=Disabled  DerivativeFilterVariant=ContFilter  NVariant=InternalParameters  NCopyVariant=Disabled  FilterICVariant=InternalICsFilter  IntegratorICVariant=Disabled  ExternalResetVariant=Disabled  TRSumVariant=Passthrough  SumFdbkVariant=Disabled  SumVariant=Sum_PD  TsampFilterVariant=InternalTs  TsampNgainVariant=Passthrough  TsampIntegralVariant=Disabled_SignalSpec  ExternalSaturationOutDataTypeStr=Inherit: Same as second input
      settings: SourceProductBaseCode=SL
  C_q2 : pid_lib/PID Controller (2DOF)  Controller=PD  Form=Parallel  TimeDomain=Continuous-time  UseExternalTs=off  SampleTime=-1  IntegratorMethod=Forward Euler  FilterMethod=Forward Euler  ControllerParametersSource=internal  P=Kp_grav  I=307.702571204868  D=Kd_grav  UseFilter=on  N=N  b=1  c=1  TunerSelectOption=Transfer Function Based (PID Tuner App)  InitialConditionSource=internal  InitialConditionForIntegrator=0  InitialConditionForFilter=0  DifferentiatorICPrevScaledInput=0  ExternalReset=none  TrackingMode=off  Kt=1  LimitOutput=off  SatLimitsSource=internal  UpperSaturationLimit=inf  LowerSaturationLimit=-inf  LinearizeAsGain=on  AntiWindupMode=none  Kb=1  POutMin=[]  POutMax=[]  IOutMin=[]  IOutMax=[]  DOutMin=[]  DOutMax=[]  NOutMin=[]  NOutMax=[]  bOutMin=[]  bOutMax=[]  cOutMin=[]  cOutMax=[]  SumOutMin=[]  SumOutMax=[]  SaturationOutMin=[]  SaturationOutMax=[]  PParamMin=[]  PParamMax=[]  IParamMin=[]  IParamMax=[]  DParamMin=[]  DParamMax=[]  NParamMin=[]  NParamMax=[]  bParamMin=[]  bParamMax=[]  cParamMin=[]  cParamMax=[]  KbParamMin=[]  KbParamMax=[]  KtParamMin=[]  KtParamMax=[]  KbOutMin=[]  KbOutMax=[]  KtOutMin=[]  KtOutMax=[]  IntegratorOutMin=[]  IntegratorOutMax=[]  FilterOutMin=[]  FilterOutMax=[]  SumI1OutMin=[]  SumI1OutMax=[]  SumI2OutMin=[]  SumI2OutMax=[]  SumI3OutMin=[]  SumI3OutMax=[]  SumI4OutMin=[]  SumI4OutMax=[]  SumDOutMin=[]  SumDOutMax=[]  Sum1OutMin=[]  Sum1OutMax=[]  Sum2OutMin=[]  Sum2OutMax=[]  Sum3OutMin=[]  Sum3OutMax=[]  DifferentiatorOutMin=[]  DifferentiatorOutMax=[]  FilterDiffOutCoefMin=[]  FilterDiffOutCoefMax=[]  ReciprocalOutMin=[]  ReciprocalOutMax=[]  SumDenOutMin=[]  SumDenOutMax=[]  SumNumOutMin=[]  SumNumOutMax=[]  DivideOutMin=[]  DivideOutMax=[]  UdiffTsProdOutMin=[]  UdiffTsProdOutMax=[]  NTsProdOutMin=[]  NTsProdOutMax=[]  UintegralTsProdOutMin=[]  UintegralTsProdOutMax=[]  UngainTsProdOutMin=[]  UngainTsProdOutMax=[]  IntegratorContinuousStateAttributes=''  IntegratorStateMustResolveToSignalObject=off  IntegratorRTWStateStorageClass=Auto  FilterContinuousStateAttributes=''  FilterStateMustResolveToSignalObject=off  FilterRTWStateStorageClass=Auto  ParallelPVariant=InternalParameters  IdealPVariant=Disabled  IVariant=Disabled  DVariant=InternalParameters  bVariant=InternalParameters  cVariant=InternalParameters  IntegratorVariant=Disabled  SatVariant=Disabled  AWVariant=Disabled  PCopyVariant=Disabled  TRVariant=Disabled  FdbkBlocksVariant=Forward  IdealPFdbkVariant=Disabled  SatFdbkVariant=Disabled  DerivativeFilterVariant=ContFilter  NVariant=InternalParameters  NCopyVariant=Disabled  FilterICVariant=InternalICsFilter  IntegratorICVariant=Disabled  ExternalResetVariant=Disabled  TRSumVariant=Passthrough  SumFdbkVariant=Disabled  SumVariant=Sum_PD  TsampFilterVariant=InternalTs  TsampNgainVariant=Passthrough  TsampIntegralVariant=Disabled_SignalSpec  ExternalSaturationOutDataTypeStr=Inherit: Same as second input
      settings: SourceProductBaseCode=SL
  Constant16 : Constant  Value=m1
  Constant17 : Constant  Value=g
  Constant18 : Constant  Value=m2
  Constant19 : Constant  Value=L1x
  Constant2 : Constant  Value=L2x
  Demux : Demux  Outputs=2
  Gain{1..5} (5 alike) : Gain  Gain=param_dev
  Gravity compensation : MATLAB Function  TreatAsAtomicUnit=on
  Mux2 : Mux  Inputs=2
  Sum{,1..3} (4 alike) : Sum  Inputs=++|
  tau : Outport
  wires:
  Mux2/1 -> tau/1
  Sum/1 -> Mux2/1
  Sum1/1 -> Mux2/2
  q_cmd_bus/1 -> [CMD]
  plant_bus/1 -> [PLANT]
  Demux/1 -> Sum/1
  Demux/2 -> Sum1/1
  C_q2/1 -> Sum2/2
  [CMD] -> Bus Selector7/1, Bus Selector3/1, Bus Selector/1
  [PLANT] -> Bus Selector2/1, Bus Selector1/1
  Bus Selector1/1 -> C_q1/2  "<q1>"
  Bus Selector2/1 -> C_q2/2  "<q2>"
  Bus Selector3/1 -> C_q2/1  "<cmd_q2>"
  Bus Selector/1 -> C_q1/1  "<cmd_q1>"
  C_q1/1 -> Sum3/2
  Sum3/1 -> Sum/2
  Sum2/1 -> Sum1/2
  Bus Selector7/1 -> Sum3/1  "<cmd_q1_dd>"
  Bus Selector7/2 -> Sum2/1  "<cmd_q2_dd>"
  Gain2/1 -> Gravity compensation/3(g)
  Gain5/1 -> Gravity compensation/5(m2)
  Bus Selector5/2 -> Gravity compensation/7(q2)  "<q2>"
  Constant18/1 -> Gain5/1
  [PLANT] -> Bus Selector5/1
  Constant2/1 -> Gain1/1
  Gravity compensation/1(G) -> Demux/1
  Constant19/1 -> Gain3/1
  Constant17/1 -> Gain2/1
  Constant16/1 -> Gain4/1
  Gain3/1 -> Gravity compensation/1(L_1x)
  Gain1/1 -> Gravity compensation/2(L_2x)
  Bus Selector5/1 -> Gravity compensation/6(q1)  "<q1>"
  Gain4/1 -> Gravity compensation/4(m1)

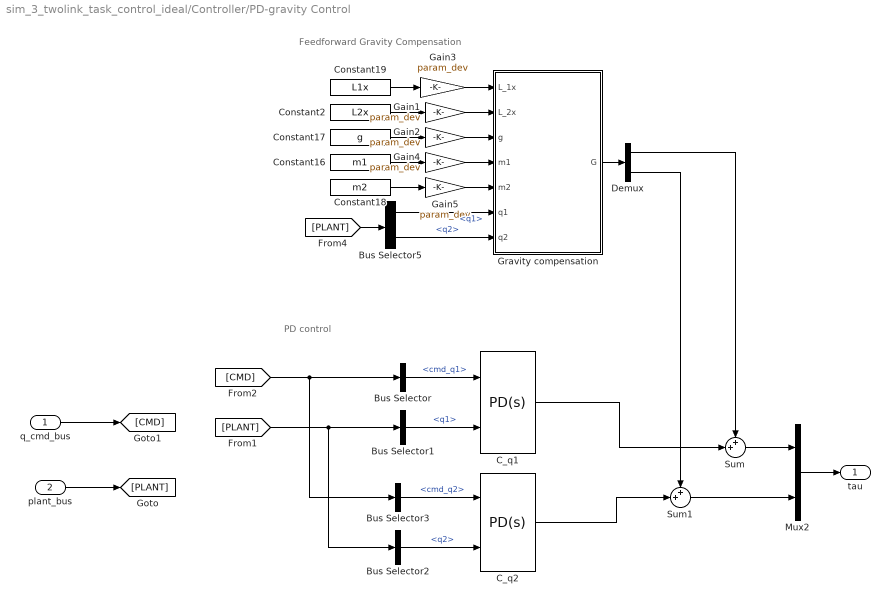
== system sim_3_twolink_task_control_ideal/Controller/PD-gravity Control  ==
  note: Feedforward Gravity Compensation
  note: PD control
  q_cmd_bus : Inport
  plant_bus : Inport  Port=2
  Bus Selector : BusSelector  OutputSignals=cmd_q1
  Bus Selector1 : BusSelector  OutputSignals=q1
  Bus Selector2 : BusSelector  OutputSignals=q2
  Bus Selector3 : BusSelector  OutputSignals=cmd_q2
  Bus Selector5 : BusSelector  OutputSignals=q1,q2
  C_q1 : pid_lib/PID Controller (2DOF)  Controller=PD  Form=Parallel  TimeDomain=Continuous-time  UseExternalTs=off  SampleTime=-1  IntegratorMethod=Forward Euler  FilterMethod=Forward Euler  ControllerParametersSource=internal  P=Kp_grav  I=20  D=Kd_grav  UseFilter=on  N=N  b=1  c=1  TunerSelectOption=Transfer Function Based (PID Tuner App)  InitialConditionSource=internal  InitialConditionForIntegrator=0  InitialConditionForFilter=0  DifferentiatorICPrevScaledInput=0  ExternalReset=none  TrackingMode=off  Kt=1  LimitOutput=off  SatLimitsSource=internal  UpperSaturationLimit=inf  LowerSaturationLimit=-inf  LinearizeAsGain=on  AntiWindupMode=none  Kb=1  POutMin=[]  POutMax=[]  IOutMin=[]  IOutMax=[]  DOutMin=[]  DOutMax=[]  NOutMin=[]  NOutMax=[]  bOutMin=[]  bOutMax=[]  cOutMin=[]  cOutMax=[]  SumOutMin=[]  SumOutMax=[]  SaturationOutMin=[]  SaturationOutMax=[]  PParamMin=[]  PParamMax=[]  IParamMin=[]  IParamMax=[]  DParamMin=[]  DParamMax=[]  NParamMin=[]  NParamMax=[]  bParamMin=[]  bParamMax=[]  cParamMin=[]  cParamMax=[]  KbParamMin=[]  KbParamMax=[]  KtParamMin=[]  KtParamMax=[]  KbOutMin=[]  KbOutMax=[]  KtOutMin=[]  KtOutMax=[]  IntegratorOutMin=[]  IntegratorOutMax=[]  FilterOutMin=[]  FilterOutMax=[]  SumI1OutMin=[]  SumI1OutMax=[]  SumI2OutMin=[]  SumI2OutMax=[]  SumI3OutMin=[]  SumI3OutMax=[]  SumI4OutMin=[]  SumI4OutMax=[]  SumDOutMin=[]  SumDOutMax=[]  Sum1OutMin=[]  Sum1OutMax=[]  Sum2OutMin=[]  Sum2OutMax=[]  Sum3OutMin=[]  Sum3OutMax=[]  DifferentiatorOutMin=[]  DifferentiatorOutMax=[]  FilterDiffOutCoefMin=[]  FilterDiffOutCoefMax=[]  ReciprocalOutMin=[]  ReciprocalOutMax=[]  SumDenOutMin=[]  SumDenOutMax=[]  SumNumOutMin=[]  SumNumOutMax=[]  DivideOutMin=[]  DivideOutMax=[]  UdiffTsProdOutMin=[]  UdiffTsProdOutMax=[]  NTsProdOutMin=[]  NTsProdOutMax=[]  UintegralTsProdOutMin=[]  UintegralTsProdOutMax=[]  UngainTsProdOutMin=[]  UngainTsProdOutMax=[]  IntegratorContinuousStateAttributes=''  IntegratorStateMustResolveToSignalObject=off  IntegratorRTWStateStorageClass=Auto  FilterContinuousStateAttributes=''  FilterStateMustResolveToSignalObject=off  FilterRTWStateStorageClass=Auto  ParallelPVariant=InternalParameters  IdealPVariant=Disabled  IVariant=Disabled  DVariant=InternalParameters  bVariant=InternalParameters  cVariant=InternalParameters  IntegratorVariant=Disabled  SatVariant=Disabled  AWVariant=Disabled  PCopyVariant=Disabled  TRVariant=Disabled  FdbkBlocksVariant=Forward  IdealPFdbkVariant=Disabled  SatFdbkVariant=Disabled  DerivativeFilterVariant=ContFilter  NVariant=InternalParameters  NCopyVariant=Disabled  FilterICVariant=InternalICsFilter  IntegratorICVariant=Disabled  ExternalResetVariant=Disabled  TRSumVariant=Passthrough  SumFdbkVariant=Disabled  SumVariant=Sum_PD  TsampFilterVariant=InternalTs  TsampNgainVariant=Passthrough  TsampIntegralVariant=Disabled_SignalSpec  ExternalSaturationOutDataTypeStr=Inherit: Same as second input
      settings: SourceProductBaseCode=SL
  C_q2 : pid_lib/PID Controller (2DOF)  Controller=PD  Form=Parallel  TimeDomain=Continuous-time  UseExternalTs=off  SampleTime=-1  IntegratorMethod=Forward Euler  FilterMethod=Forward Euler  ControllerParametersSource=internal  P=Kp_grav  I=307.702571204868  D=Kd_grav  UseFilter=on  N=N  b=1  c=1  TunerSelectOption=Transfer Function Based (PID Tuner App)  InitialConditionSource=internal  InitialConditionForIntegrator=0  InitialConditionForFilter=0  DifferentiatorICPrevScaledInput=0  ExternalReset=none  TrackingMode=off  Kt=1  LimitOutput=off  SatLimitsSource=internal  UpperSaturationLimit=inf  LowerSaturationLimit=-inf  LinearizeAsGain=on  AntiWindupMode=none  Kb=1  POutMin=[]  POutMax=[]  IOutMin=[]  IOutMax=[]  DOutMin=[]  DOutMax=[]  NOutMin=[]  NOutMax=[]  bOutMin=[]  bOutMax=[]  cOutMin=[]  cOutMax=[]  SumOutMin=[]  SumOutMax=[]  SaturationOutMin=[]  SaturationOutMax=[]  PParamMin=[]  PParamMax=[]  IParamMin=[]  IParamMax=[]  DParamMin=[]  DParamMax=[]  NParamMin=[]  NParamMax=[]  bParamMin=[]  bParamMax=[]  cParamMin=[]  cParamMax=[]  KbParamMin=[]  KbParamMax=[]  KtParamMin=[]  KtParamMax=[]  KbOutMin=[]  KbOutMax=[]  KtOutMin=[]  KtOutMax=[]  IntegratorOutMin=[]  IntegratorOutMax=[]  FilterOutMin=[]  FilterOutMax=[]  SumI1OutMin=[]  SumI1OutMax=[]  SumI2OutMin=[]  SumI2OutMax=[]  SumI3OutMin=[]  SumI3OutMax=[]  SumI4OutMin=[]  SumI4OutMax=[]  SumDOutMin=[]  SumDOutMax=[]  Sum1OutMin=[]  Sum1OutMax=[]  Sum2OutMin=[]  Sum2OutMax=[]  Sum3OutMin=[]  Sum3OutMax=[]  DifferentiatorOutMin=[]  DifferentiatorOutMax=[]  FilterDiffOutCoefMin=[]  FilterDiffOutCoefMax=[]  ReciprocalOutMin=[]  ReciprocalOutMax=[]  SumDenOutMin=[]  SumDenOutMax=[]  SumNumOutMin=[]  SumNumOutMax=[]  DivideOutMin=[]  DivideOutMax=[]  UdiffTsProdOutMin=[]  UdiffTsProdOutMax=[]  NTsProdOutMin=[]  NTsProdOutMax=[]  UintegralTsProdOutMin=[]  UintegralTsProdOutMax=[]  UngainTsProdOutMin=[]  UngainTsProdOutMax=[]  IntegratorContinuousStateAttributes=''  IntegratorStateMustResolveToSignalObject=off  IntegratorRTWStateStorageClass=Auto  FilterContinuousStateAttributes=''  FilterStateMustResolveToSignalObject=off  FilterRTWStateStorageClass=Auto  ParallelPVariant=InternalParameters  IdealPVariant=Disabled  IVariant=Disabled  DVariant=InternalParameters  bVariant=InternalParameters  cVariant=InternalParameters  IntegratorVariant=Disabled  SatVariant=Disabled  AWVariant=Disabled  PCopyVariant=Disabled  TRVariant=Disabled  FdbkBlocksVariant=Forward  IdealPFdbkVariant=Disabled  SatFdbkVariant=Disabled  DerivativeFilterVariant=ContFilter  NVariant=InternalParameters  NCopyVariant=Disabled  FilterICVariant=InternalICsFilter  IntegratorICVariant=Disabled  ExternalResetVariant=Disabled  TRSumVariant=Passthrough  SumFdbkVariant=Disabled  SumVariant=Sum_PD  TsampFilterVariant=InternalTs  TsampNgainVariant=Passthrough  TsampIntegralVariant=Disabled_SignalSpec  ExternalSaturationOutDataTypeStr=Inherit: Same as second input
      settings: SourceProductBaseCode=SL
  Constant16 : Constant  Value=m1
  Constant17 : Constant  Value=g
  Constant18 : Constant  Value=m2
  Constant19 : Constant  Value=L1x
  Constant2 : Constant  Value=L2x
  Demux : Demux  Outputs=2
  Gain{1..5} (5 alike) : Gain  Gain=param_dev
  Gravity compensation : MATLAB Function  TreatAsAtomicUnit=on
  Mux2 : Mux  Inputs=2
  Sum : Sum  Inputs=++|
  Sum1 : Sum  Inputs=++|
  tau : Outport
  wires:
  Mux2/1 -> tau/1
  Sum/1 -> Mux2/1
  Sum1/1 -> Mux2/2
  q_cmd_bus/1 -> [CMD]
  plant_bus/1 -> [PLANT]
  Constant19/1 -> Gain3/1
  Constant18/1 -> Gain5/1
  Constant2/1 -> Gain1/1
  Constant16/1 -> Gain4/1
  Constant17/1 -> Gain2/1
  Bus Selector5/1 -> Gravity compensation/6(q1)  "<q1>"
  [PLANT] -> Bus Selector5/1
  Bus Selector5/2 -> Gravity compensation/7(q2)  "<q2>"
  Gravity compensation/1(G) -> Demux/1
  Demux/1 -> Sum/1
  Demux/2 -> Sum1/1
  C_q2/1 -> Sum1/2
  [CMD] -> Bus Selector3/1, Bus Selector/1
  [PLANT] -> Bus Selector2/1, Bus Selector1/1
  Bus Selector1/1 -> C_q1/2  "<q1>"
  Bus Selector2/1 -> C_q2/2  "<q2>"
  Bus Selector3/1 -> C_q2/1  "<cmd_q2>"
  Bus Selector/1 -> C_q1/1  "<cmd_q1>"
  C_q1/1 -> Sum/2
  Gain3/1 -> Gravity compensation/1(L_1x)
  Gain1/1 -> Gravity compensation/2(L_2x)
  Gain2/1 -> Gravity compensation/3(g)
  Gain4/1 -> Gravity compensation/4(m1)
  Gain5/1 -> Gravity compensation/5(m2)
